simulink model "check_TorqueRequest"  (R2018b)
settings: configuration reference "Physics" (kept outside this file)
model workspace (MAT data in the model file):
  veh_param = Simulink.Parameter
  veh_param.Value.cLiftF = 0
  veh_param.Value.cLiftR = 0
  veh_param.Value.CoGx_m = 0
  veh_param.Value.CoGy_m = 0
  veh_param.Value.CoGz_m = 0
  veh_param.Value.cDrag = 0
  veh_param.Value.Aref_m2 = 0
  veh_param.Value.Gearratio = 0
  veh_param.Value.Wheelbase_m = 0
  veh_param.Value.PacLatF = [0 0 0 0 0]
  veh_param.Value.PacLongF = [0 0 0 0 0]
  veh_param.Value.PacLatR = [0 0 0 0 0]
  veh_param.Value.PacLongR = [0 0 0 0 0]
  veh_param.Value.cRollFriction_Npmps = 0
  veh_param.Value.MaxRollFriction_N = 0
  veh_param.Value.T_YawRate_s = 0
  veh_param.Value.T_LatVel_s = 0
  veh_param.Value.TrackWidthF_m = 0
  veh_param.Value.TrackWidthR_m = 0
  veh_param.Value.TireRadiusF_m = 0
  veh_param.Value.TireRadiusR_m = 0
  veh_param.Value.VehicleInertia_kgm2 = 0
  veh_param.Value.WheelInertiaF_kgm2 = 0
  veh_param.Value.WheelInertiaR_kgm2 = 0
  veh_param.Value.VehicleMass_kg = 0
  veh_param.Value.switchModelBlend_mps = 0
  veh_param.Value.PTLimitLowVel_N = 0
  veh_param.Value.switchModelVel_mps = 0
  veh_param.Value.T_Tire_s = 0
  veh_param.DataType = 'struct'
  veh_param.Dimensions = [1 1]
  x0_positionstates = Simulink.Parameter
  x0_positionstates.Value = [0 0 0]
  x0_positionstates.DataType = 'auto'
  x0_positionstates.Dimensions = [1 3]
libraries: simulink x1
settings Model: DataDictionary=vehicleparameters_vehdynsim.sldd  OrderedModelArguments=off  Creator=wischnewski  LastModifiedBy=ga25xiw

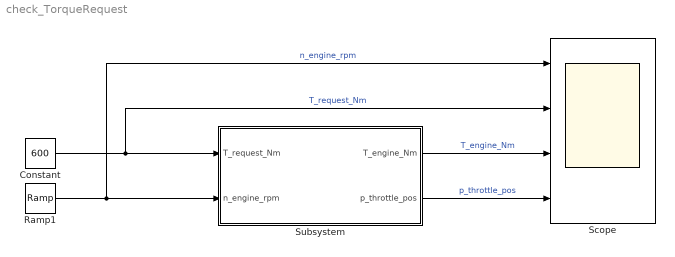
== system check_TorqueRequest ==
  Constant : Constant  Value=600
  Ramp1 : simulink/Sources/Ramp  slope=700  start=0  InitialOutput=0
  Scope : Scope  NumInputPorts=4
  Subsystem : Subsystem
  wires:
  Constant/1 -> Subsystem/1(T_request_Nm), Scope/2  "T_request_Nm"
  Ramp1/1 -> Subsystem/2(n_engine_rpm), Scope/1  "n_engine_rpm"
  Subsystem/2(p_throttle_pos) -> Scope/4  "p_throttle_pos"
  Subsystem/1(T_engine_Nm) -> Scope/3  "T_engine_Nm"

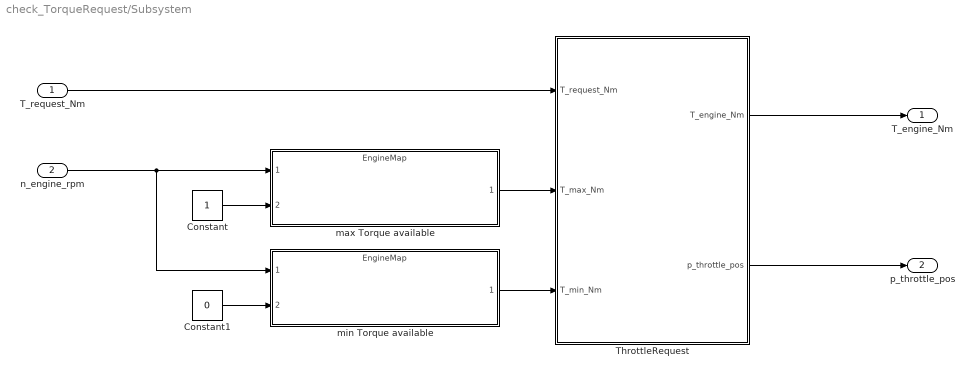
== system check_TorqueRequest/Subsystem ==
  T_request_Nm : Inport
  n_engine_rpm : Inport  Port=2
  Constant : Constant
  Constant1 : Constant  Value=0
  ThrottleRequest : MATLAB Function  TreatAsAtomicUnit=on
  max Torque available : ModelReference  ModelNameDialog=EngineMap.slx  SimulationMode=Normal  ModelReferenceVersion=1.393
  min Torque available : ModelReference  ModelNameDialog=EngineMap.slx  SimulationMode=Normal  ModelReferenceVersion=1.393
  T_engine_Nm : Outport
  p_throttle_pos : Outport  Port=2
  wires:
  ThrottleRequest/2(p_throttle_pos) -> p_throttle_pos/1
  min Torque available/1 -> ThrottleRequest/3(T_min_Nm)
  Constant1/1 -> min Torque available/2
  Constant/1 -> max Torque available/2
  T_request_Nm/1 -> ThrottleRequest/1(T_request_Nm)
  max Torque available/1 -> ThrottleRequest/2(T_max_Nm)
  n_engine_rpm/1 -> min Torque available/1, max Torque available/1
  ThrottleRequest/1(T_engine_Nm) -> T_engine_Nm/1

== matlab function check_TorqueRequest/Subsystem/ThrottleRequest ==
  data: T_request_Nm input; T_engine_Nm output; T_max_Nm input; T_min_Nm input; p_throttle_pos output
function [T_engine_Nm, p_throttle_pos] = fcn(T_request_Nm, T_max_Nm, T_min_Nm)

[T_engine_Nm, p_throttle_pos] = ThrottleRequest(T_request_Nm, T_max_Nm, T_min_Nm);
